simulink model "controller"  (R2020b)
settings: Solver=VariableStepAuto  StartTime=0.0  StopTime=100  MaxStep=0.01  RelTol=1e-3
values from neighbouring files (symbols this model uses):
  fi_dot_des = 0    [params.m]
  J = 1    [params.m]
  k_p_fi = 0.1    [params.m]
  k_p_x = 0.1    [params.m]
  k_p_y = 0.1    [params.m]
  k_v_fi = 0.5    [params.m]
  k_v_x = 0.5    [params.m]
  k_v_y = 0.5    [params.m]
  m = 1    [params.m]
  x_des = 6    [params.m]
  x_dot_des = 0    [params.m]
  y_des = 4    [params.m]
  y_dot_des = 0    [params.m]
libraries: simulink_extras x2
settings Model: Creator=Danil  LastModifiedBy=Danil

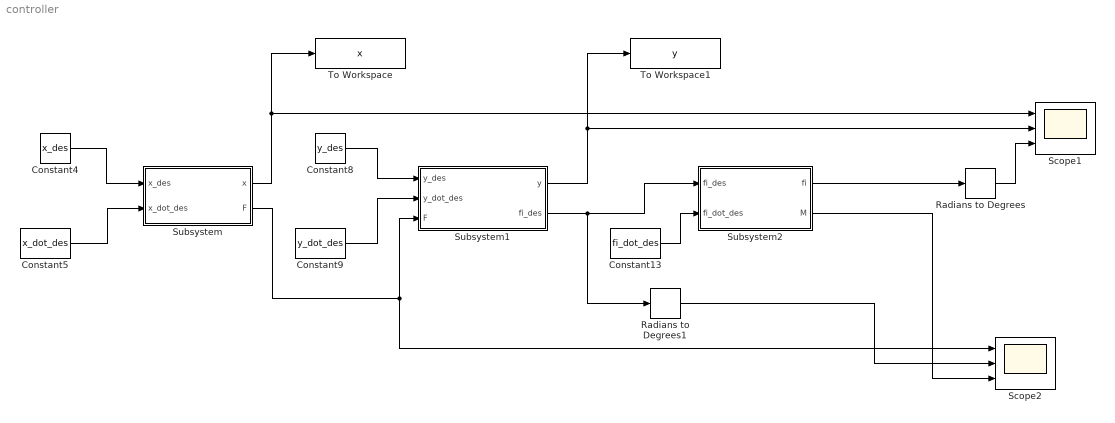
== system controller ==
  Constant13 : Constant  Value=fi_dot_des
  Constant4 : Constant  Value=x_des
  Constant5 : Constant  Value=x_dot_des
  Constant8 : Constant  Value=y_des
  Constant9 : Constant  Value=y_dot_des
  Radians to Degrees : simulink_extras/Transformations/Radians to Degrees
  Radians to Degrees1 : simulink_extras/Transformations/Radians to Degrees
  Scope1 : Scope  NumInputPorts=3
  Scope2 : Scope  NumInputPorts=3
  Subsystem : Subsystem
  Subsystem1 : Subsystem
  Subsystem2 : Subsystem
  To Workspace : ToWorkspace  VariableName=x  SaveFormat=Timeseries  SampleTime=-1
  To Workspace1 : ToWorkspace  VariableName=y  SaveFormat=Timeseries  SampleTime=-1
  wires:
  Radians to Degrees/1 -> Scope1/3
  Radians to Degrees1/1 -> Scope2/2
  Subsystem/2(F) -> Scope2/1, Subsystem1/3(F)
  Subsystem/1(x) -> To Workspace/1, Scope1/1
  Constant4/1 -> Subsystem/1(x_des)
  Constant5/1 -> Subsystem/2(x_dot_des)
  Subsystem1/1(y) -> To Workspace1/1, Scope1/2
  Subsystem1/2(fi_des) -> Subsystem2/1(fi_des), Radians to Degrees1/1
  Constant8/1 -> Subsystem1/1(y_des)
  Constant9/1 -> Subsystem1/2(y_dot_des)
  Constant13/1 -> Subsystem2/2(fi_dot_des)
  Subsystem2/1(fi) -> Radians to Degrees/1
  Subsystem2/2(M) -> Scope2/3

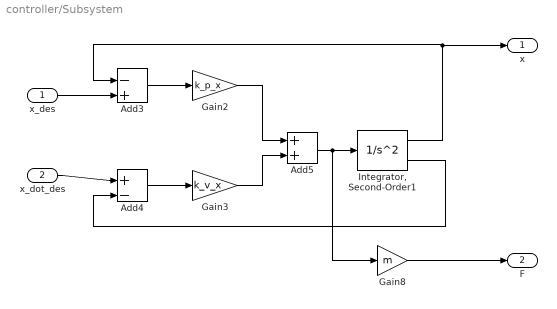
== system controller/Subsystem ==
  x_des : Inport
  x_dot_des : Inport  Port=2
  Add3 : Sum  Inputs=-|+
  Add4 : Sum  Inputs=+|-
  Add5 : Sum
  Gain2 : Gain  Gain=k_p_x
  Gain3 : Gain  Gain=k_v_x
  Gain8 : Gain  Gain=m
  "Integrator, Second-Order1" : SecondOrderIntegrator
  x : Outport
  F : Outport  Port=2
  wires:
  Add5/1 -> Gain8/1, "Integrator, Second-Order1"/1
  "Integrator, Second-Order1"/2 -> Add4/2
  Gain2/1 -> Add5/1
  x_dot_des/1 -> Add4/1
  "Integrator, Second-Order1"/1 -> Add3/1, x/1
  Add4/1 -> Gain3/1
  Gain3/1 -> Add5/2
  Gain8/1 -> F/1
  Add3/1 -> Gain2/1
  x_des/1 -> Add3/2

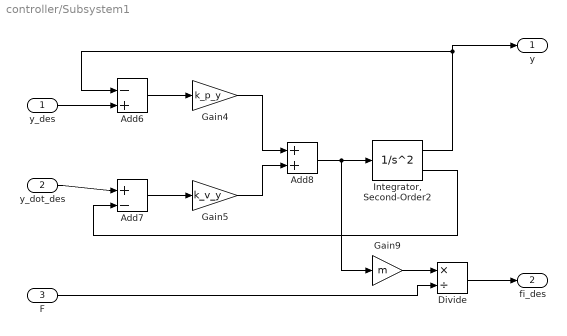
== system controller/Subsystem1 ==
  y_des : Inport
  y_dot_des : Inport  Port=2
  F : Inport  Port=3
  Add6 : Sum  Inputs=-|+
  Add7 : Sum  Inputs=+|-
  Add8 : Sum
  Divide : Product  Inputs=*/
  Gain4 : Gain  Gain=k_p_y
  Gain5 : Gain  Gain=k_v_y
  Gain9 : Gain  Gain=m
  "Integrator, Second-Order2" : SecondOrderIntegrator
  y : Outport
  fi_des : Outport  Port=2
  wires:
  Add7/1 -> Gain5/1
  Add6/1 -> Gain4/1
  "Integrator, Second-Order2"/2 -> Add7/2
  Add8/1 -> Gain9/1, "Integrator, Second-Order2"/1
  Gain4/1 -> Add8/1
  Gain5/1 -> Add8/2
  "Integrator, Second-Order2"/1 -> y/1, Add6/1
  y_des/1 -> Add6/2
  Gain9/1 -> Divide/1
  y_dot_des/1 -> Add7/1
  Divide/1 -> fi_des/1
  F/1 -> Divide/2

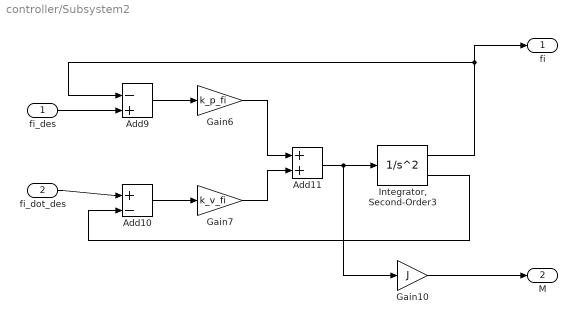
== system controller/Subsystem2 ==
  fi_des : Inport
  fi_dot_des : Inport  Port=2
  Add10 : Sum  Inputs=+|-
  Add11 : Sum
  Add9 : Sum  Inputs=-|+
  Gain10 : Gain  Gain=J
  Gain6 : Gain  Gain=k_p_fi
  Gain7 : Gain  Gain=k_v_fi
  "Integrator, Second-Order3" : SecondOrderIntegrator
  fi : Outport
  M : Outport  Port=2
  wires:
  fi_dot_des/1 -> Add10/1
  "Integrator, Second-Order3"/1 -> fi/1, Add9/1
  Add11/1 -> Gain10/1, "Integrator, Second-Order3"/1
  Add10/1 -> Gain7/1
  "Integrator, Second-Order3"/2 -> Add10/2
  Add9/1 -> Gain6/1
  Gain10/1 -> M/1
  Gain6/1 -> Add11/1
  Gain7/1 -> Add11/2
  fi_des/1 -> Add9/2
